simulink model "controller_stateflow"  (R2022b)
settings: Solver=FixedStepAuto  StartTime=0.0  StopTime=inf  FixedStep=0.05  RelTol=1e-3
PreLoadFcn:
  | rosinit();
model workspace (MAT data in the model file):
  SL_ROS_VariableLengthArrays_MaxSizes : object (value not decoded)
  pitch = -10
  restart = 0
undefined symbols (not defined in the file): StartTime
libraries: robotmaniplib x62, robotlib x17, robotcorelib x4, robotgazebolib x1
(part 2 of 4)

== system controller_stateflow/Summit Controller Command ==
  time : Inport
  sum_cntr : Inport  Port=2
  Enable : EnablePort
  Blank Message4 : robotlib/Blank Message  messageClass=Message  entityType=geometry_msgs/Twist  messageType=geometry_msgs/Twist  SampleTime=inf  legacyBusStruct=off
  Publish : robotlib/Publish  topicSource=Select from ROS network  topic=/robotnik_base_control/cmd_vel  messageType=geometry_msgs/Twist  legacyBusStruct=off  messageQueueLength=1
  summit_VelocityController_command : MATLAB Function  TreatAsAtomicUnit=on
  wires:
  Blank Message4/1 -> summit_VelocityController_command/2(msgIn)
  summit_VelocityController_command/1(msgOut) -> Publish/1
  time/1 -> summit_VelocityController_command/1(Time)
  sum_cntr/1 -> summit_VelocityController_command/3(sum_cntr)

== system controller_stateflow/UR10e Controller Command ==
  time : Inport
  TimeFromStart : Inport  Port=2
  Point_array : Inport  Port=3
  Enable : EnablePort
  Blank Message : robotlib/Blank Message  messageClass=Message  entityType=trajectory_msgs/JointTrajectory  messageType=trajectory_msgs/JointTrajectory  SampleTime=inf  legacyBusStruct=off
  Blank Message1 : robotlib/Blank Message  messageClass=Message  entityType=trajectory_msgs/JointTrajectoryPoint  messageType=trajectory_msgs/JointTrajectoryPoint  SampleTime=inf  legacyBusStruct=off
  Publish : robotlib/Publish  topicSource=Select from ROS network  topic=/ur10e_eff_joint_traj_controller/command  messageType=trajectory_msgs/JointTrajectory  legacyBusStruct=off  messageQueueLength=1
  ur10e_TrajectoryController_command : MATLAB Function  TreatAsAtomicUnit=on
  wires:
  Blank Message/1 -> ur10e_TrajectoryController_command/2(msgIn)
  Blank Message1/1 -> ur10e_TrajectoryController_command/3(msgPoint)
  ur10e_TrajectoryController_command/1(msgOut) -> Publish/1
  time/1 -> ur10e_TrajectoryController_command/1(Time)
  TimeFromStart/1 -> ur10e_TrajectoryController_command/4(TimeFromStart)
  Point_array/1 -> ur10e_TrajectoryController_command/5(Point_array)

== matlab function controller_stateflow/General State Flow/get_panda_pose3/MATLAB Function ==
  data: Pose output; boxPos input; boxZYX input; sumPos input; sumZYX input; panda_state input; Weights output; initialGuess output; state input; NWayPoints output; durTime output
function [Pose, Weights, initialGuess, NWayPoints, durTime] = fcn(boxPos,boxZYX,sumPos,sumZYX,panda_state,state)
    
    distance_10 = 0.2;
    distance_10_h = 0.1;

    dimBox   = [0.2;0.2;0.13]; %like a box but we know it's a cilinder
    dimboxUp = [0.23;0.23;0.03]; 
    box_center = [0.115;0.115;0.065]; %to mach the origin of stl with real 3D origin of the cilinder

    toSumChapa = [0;0;0.51];
    toFranka = [0.25;-0.22+0.02;0.15];
    boxPos_offset = [0;0;0];
    
    NWayPoints = 1;
    durTime = 2;
    distance = eye(4,4);
    ZYX_d = [0,0,0];

    Weights = [1,1,1,1,1,1];


    if state == 2
        boxPos_offset = [0;dimBox(2)/2+0.05;+dimBox(3)/2]+box_center;
        ZYX_d = [pi+pi/2,-pi/2,0];
        distance = [[eul2rotm([0,0,0],'ZYX')],[-distance_10,0,0]'; ...
                                0 0 0                       1              ];
        NWayPoints = 1;
        durTime = 2;
    end
    if state == 4
        boxPos_offset = [0;dimBox(2)/2+0.05;+dimBox(3)/2-0.1]+box_center;
        ZYX_d = [pi+pi/2,-pi/2,0];
        distance = [[eul2rotm([0,0,0],'ZYX')],[0,0,0]'; ...
                                0 0 0            1   ];
        NWayPoints = 3;
        durTime = 2;
    end
    if state == 5
        boxPos_offset = [0;dimBox(2)/2;+dimBox(3)/2-0.1]+box_center;
        ZYX_d = [pi+pi/2,-pi/2,0];
        NWayPoints = 5;
        durTime = 2;
    end
    if state == 6
        boxPos_offset = [0;dimBox(2)/2-0.02;+dimBox(3)/2-0.03]+box_center;
        ZYX_d = [pi+pi/2,-pi/2,0];
        NWayPoints = 5;
        durTime = 2;
    end
    if state == 9
        boxPos_offset = [0;dimBox(2)/2;+dimBox(3)/2]+box_center;
        distance = [[eul2rotm([0,0,0],'ZYX')],[-0.15,0,+0.1]'; ...
                        0 0 0            1   ];
        ZYX_d = [pi/2,0,0];
        NWayPoints = 5;
        durTime = 2;
    end
    if state == 11
        boxPos_offset = [0;dimBox(2)/2+0.02;dimBox(3)/2-0.02]+box_center;
        ZYX_d = [pi+pi/2,-pi/16,0];
        boxPos =[1;0;0.65];     %pose in terna summit::base_footprint
        boxZYX =[-pi/2;0;0];
        sumPos = [0;0;0];
        sumZYX = [0;0;0];
        NWayPoints = 5;
        durTime = 5;
    end

    if state == 12
        boxPos_offset = [0;-dimBox(2)/2-0.12;+dimBox(3)/2+0.07]+box_center;
        ZYX_d = [pi/2,-pi/16,0];
        NWayPoints = 5;
        durTime = 5;
    end

    if state == 13
        boxPos_offset = [0;-dimBox(2)/2-0.09;+dimBox(3)/2-0.02]+box_center;
        ZYX_d = [pi/2,-pi/16,0];
        NWayPoints = 5;
        durTime = 5;
    end

    % Trasformazione world -> box::frame
    boxtf_01 = [[eul2rotm(boxZYX', 'ZYX')],boxPos; ...
            0 0 0                               1           ];
    % Trasformazione world -> summit::base_footprint
    sumtf_01 = [[eul2rotm(sumZYX', 'ZYX')],sumPos; ...
                0 0 0                               1           ];
    
    % Trasformazione summit::base_footprint -> panda::base
    sumtopandatf_12 = [[eul2rotm([0,pi/4,0], 'ZYX')],toSumChapa+toFranka; ...
                0 0 0                               1           ];
    
    % Trasformazione world -> panda::base
    toPandatf = sumtf_01*sumtopandatf_12;
    
    % Trasformo la posizione da world frame a panda::base frame per l'IK
    Pose_d0 = boxtf_01*[[eul2rotm(ZYX_d,'ZYX')],[boxPos_offset(1);boxPos_offset(2);boxPos_offset(3)]; ...
                                0 0 0                               1           ];

    Pose = distance*inv(toPandatf)*Pose_d0;

    initialGuess = panda_state;

end

== matlab function controller_stateflow/General State Flow/get_ur_pose_cnvy/MATLAB Function3 ==
  data: u input; y output
function y = fcn(u)

y = u(1:6);

== matlab function controller_stateflow/General State Flow/get_panda_pose3/MATLAB Function4 ==
  data: pose_d input; Pose1 output; T input; Pose2 output; Pose3 output; NWayPoint input; Pose4 output; Pose5 output
function [Pose1,Pose2,Pose3,Pose4,Pose5] = fcn(pose_d,T,NWayPoint)

    coder.extrinsic('slerp');

    if NWayPoint == 1
        Pose1 = pose_d;
        Pose2 = pose_d;
        Pose3 = pose_d;
        Pose4 = pose_d;
        Pose5 = pose_d;
    else

        %semplice interpolazione lineare sulla posizione tra posizione
        %attuale e posizione desiderata
        pos_act   = T(1:3,4);
        pos_d     = pose_d(1:3,4);
        delta_pos = (pos_d-pos_act)/5; 
                  
        q_d = rotm2quat(pose_d(1:3,1:3));
        q_a = rotm2quat(T(1:3,1:3));
        q =   slerp(quaternion(q_a),quaternion(q_d),0:0.2:1);

        Pose1 = [quat2rotm(q(1)),pos_act+delta_pos*1; ...
                 0 0 0                               1           ];
        Pose2 = [quat2rotm(q(2)),pos_act+delta_pos*2; ...
                 0 0 0                               1           ];
        Pose3 = [quat2rotm(q(3)),pos_act+delta_pos*3; ...
                 0 0 0                               1           ];
        Pose4 = [quat2rotm(q(4)),pos_act+delta_pos*4; ...
                 0 0 0                               1           ];

        Pose5 = pose_d;
    end

end

== matlab function controller_stateflow/Wait 0,1 second ==
  data: u input; e output double
function e = wait(u)
% Wait 1e8 nanosecond after start for all Gazebo components starting

    e=0;
    if u.Nsec > 1e8
        e=1;
    end

end

== matlab function controller_stateflow/General State Flow/get_panda_pose3/MATLAB Function6 ==
  data: u input; y output
function y = fcn(u)

y = u(1:7);

== matlab function controller_stateflow/Wait 1 second ==
  data: u input; e output double
function e = wait(u)
% Wait 1 second after start for all Gazebo components starting
    e=0;
    if u.Sec >= 1
        e=1;
    end
end

== matlab function controller_stateflow/Force Generator Function ==
  data: enable output; msgOut output Bus: SL_Bus_controller_stateflow_ApplyBodyWrenchRequest_gxwnto; msgIn input Bus: SL_Bus_controller_stateflow_ApplyBodyWrenchRequest_gxwnto; state input; coll input; T_ur_velvCnt input; pick_type input; state_4_collBox input
function [enable,msgOut]  = force_generator(msgIn,state,coll,T_ur_velvCnt, pick_type, state_4_collBox)

    msgOut = msgIn;
    
    bodyname = 'box_38_18_14::link_0';   % type 1
  
    if pick_type == 1
        bodyname = 'box_38_18_14::link_0';
        else if pick_type == 2
                bodyname = 'box_19_14_29::link_0';
            else if pick_type == 3
                    bodyname = 'cilinder_20_13::link_0';
                else if pick_type == 4 && state_4_collBox == 1
                        bodyname = 'box_38_18_14::link_0';
                    else if pick_type == 4 && state_4_collBox == 2
                        bodyname = 'box_38_18_14_0::link_0';
                    end
                end
            end
        end
    end

    enable = 0;
    
    lenName = uint32(length(bodyname));
    msgOut.BodyName(1:lenName,1) = uint8(convertStringsToChars(bodyname))';
    msgOut.BodyName_SL_Info.CurrentLength = uint32(lenName);
   
    msgOut.ReferenceFrame(1:lenName,1) = uint8(convertStringsToChars(bodyname))';
    msgOut.ReferenceFrame_SL_Info.CurrentLength = uint32(lenName);
    
    msgOut.Wrench.Force.X =  0;
    msgOut.Wrench.Force.Y =  0;
    msgOut.Wrench.Force.Z =  0;
    msgOut.Wrench.Torque.X = 0;
    msgOut.Wrench.Torque.Y = 0;
    msgOut.Wrench.Torque.Z = 0;
        
    F_v = [0;0;0;1];

    if state == 1 && coll == 1
        k=0.75;
%         F_v = [0;0;-80*k;1];
        F_v = [-80*k;0;0;1];

        msgOut.Wrench.Torque.X = 0;
        msgOut.Wrench.Torque.Y = 0;
        msgOut.Wrench.Torque.Z = 0;

        msgOut.ReferencePoint.X = 0;
        msgOut.ReferencePoint.Y = 0;
        msgOut.ReferencePoint.Z = 0;
        
        msgOut.Duration.Sec = 0;
        msgOut.Duration.Nsec = 1e7;

        fprintf("pull \n");

        enable = 1;
    end


    if state == -1
        k=1.0;
%         F_v = [0;0;80*k;1];
        F_v = [80*k;0;0;1];

        msgOut.Wrench.Torque.X = 0;
        msgOut.Wrench.Torque.Y = 0;
        msgOut.Wrench.Torque.Z = 0;
        
        msgOut.ReferencePoint.X = 0;
        msgOut.ReferencePoint.Y = 0;
        msgOut.ReferencePoint.Z = 0;

        msgOut.Duration.Sec = 0;
        msgOut.Duration.Nsec = 1e7;

        fprintf("push \n");

        enable = 1;        
    end
        
    F_w = T_ur_velvCnt*F_v;

    msgOut.Wrench.Force.X = F_w(1);
    msgOut.Wrench.Force.Y = F_w(2);
    msgOut.Wrench.Force.Z = F_w(3);

end

== matlab function controller_stateflow/UR10e Controller Command/ur10e_TrajectoryController_command ==
  data: Time input; msgOut output Bus: SL_Bus_controller_stateflow_trajectory_msgs_JointTrajectory; msgIn input; msgPoint input; TimeFromStart input; Point_array input
function msgOut   = ur10e_TrajectoryController_command(Time, msgIn, msgPoint,TimeFromStart, Point_array)
% In this function we create the TrajecotryJointController message for the
% ROS topic to command movements of manipulator.
    msgOut = msgIn;
    if Time.Sec ~= 0

        jointNames = {'ur10e_shoulder_pan_joint','ur10e_shoulder_lift_joint','ur10e_elbow_joint'...
            'ur10e_wrist_1_joint','ur10e_wrist_2_joint','ur10e_wrist_3_joint'};
        numJoints = uint32(length(jointNames));
        msgOut.JointNames_SL_Info.CurrentLength = numJoints;
        for idx = 1:numJoints
            jName = jointNames{idx};
            lenName = uint32(length(jName));
            msgOut.JointNames(idx).Data(1:lenName) = uint8(jName);
            msgOut.JointNames(idx).Data_SL_Info.CurrentLength = lenName;
        end

        msgOut.Header.Stamp.Sec = Time.Sec;
        msgOut.Header.Stamp.Nsec = Time.Nsec;
        
        msgOut.Header.Seq = uint32(0);
        
        %if the points are all equals, the command is to reach that point
        %in one pooint position command, in TimeFromStart time.
        if isequal(Point_array(:,1),Point_array(:,2))
            msgOut.Points_SL_Info.CurrentLength = uint32(1);
            msgOut.Points(1) = msgPoint;
            msgOut.Points(1).Positions(1:6) = Point_array(1:6,1);
            msgOut.Points(1).Positions_SL_Info.CurrentLength = uint32(6);
            msgOut.Points(1).TimeFromStart.Sec = TimeFromStart;
            msgOut.Points(1).TimeFromStart.Nsec = 0;
        else
            % otherwise the command is a trajectory command and the time is
            % divided for each point.
            msgOut.Points_SL_Info.CurrentLength = uint32(size(Point_array,2));
                
            for i = 1:size(Point_array,2)
                msgOut.Points(i) = msgPoint;
                msgOut.Points(i).Positions(1:6) = Point_array(1:6,i);
                msgOut.Points(i).Positions_SL_Info.CurrentLength = uint32(6);

                msgOut.Points(i).TimeFromStart.Sec = TimeFromStart + 1*i;
                msgOut.Points(i).TimeFromStart.Nsec = 0;

                time = TimeFromStart*1e9;
                time_i_nsec = time/5*i;
                msgOut.Points(i).TimeFromStart.Sec = fix(time_i_nsec/1e9);
                msgOut.Points(i).TimeFromStart.Nsec = time_i_nsec-fix(time_i_nsec/1e9);
            end
        end
        
    end
end

== matlab function controller_stateflow/General State Flow/get_panda_pose_cnvy/MATLAB Function ==
  data: Pose output; boxPos input; boxZYX input; sumPos input; sumZYX input; panda_state input; data input; Weights output; initialGuess output; state input; NWayPoints output; durTime output
function [Pose, Weights, initialGuess, NWayPoints, durTime] = fcn(boxPos,boxZYX,sumPos,sumZYX,panda_state,data, state)
    
    distance_10 = 0.2;
    distance_10_h = 0.1;
    dimBox=[0.38,0.18,0.14];
    toSumChapa = [0;0;0.51];
    toFranka = [0.25;-0.22+0.02;0.15];
    boxPos_offset = [0;0;0];
    
    NWayPoints = 1;
    durTime = 2;
    distance = eye(4,4);
    ZYX_d = [0,0,0];

    Weights = [1,1,1,1,1,1];


%     % Trasformazione world -> box::frame
%     boxtf_01 = [[eul2rotm(boxZYX', 'ZYX')],boxPos; ...
%             0 0 0                               1           ];
%     % Trasformazione world -> summit::base_footprint
%     sumtf_01 = [[eul2rotm(sumZYX', 'ZYX')],sumPos; ...
%                 0 0 0                               1           ];
%     
%     % Trasformazione summit::base_footprint -> panda::base
%     sumtopandatf_12 = [[eul2rotm([0,pi/4,0], 'ZYX')],toSumChapa+toFranka; ...
%                 0 0 0                               1           ];
%     
%     % Trasformazione world -> panda::base
%     toPandatf = sumtf_01*sumtopandatf_12;
%     
%     % Trasformo la posizione da world frame a panda::base frame per l'IK
%     Pose_d0 = boxtf_01*[[eul2rotm(ZYX_d,'ZYX')],[boxPos_offset(1);boxPos_offset(2);boxPos_offset(3)]; ...
%                                 0 0 0                               1           ];
% 
%     Pose = distance*inv(toPandatf)*Pose_d0;

    Pose = data + [0 0 0 0; 0 0 0 0;0 0 0 0.2;0 0 0 0];     

    initialGuess = panda_state;

end

== matlab function controller_stateflow/Collision Check/MATLAB Function4 ==
  data: x output; T input; T_end input; y output; box_pos input; box_ZYX input; box2_pos input; box2_ZYX input; z output; sumPos input; sumZYX input; T_ur_velvCnt output; coll output; boxx output; pick_type input; state_4_collBox input
function [x,y,z,T_ur_velvCnt,coll,boxx] = collision_fnc(T,T_end,box_pos,box_ZYX,box2_pos,box2_ZYX,sumPos,sumZYX,pick_type,state_4_collBox)
    
    dimBox = [0;0;0];
    box = box_pos;
    boxZYX = box_ZYX;

    % Based on the pick_type, choose the right dimensions of the box
    if pick_type == 1 || pick_type == 4
        dimBox = [0.38;0.18;0.14];
        else if pick_type == 2
                dimBox=[0.19,0.14,0.29];
            else if pick_type == 3
                    dimBox = [0.2;0.2;0.13];
                    box_center = [0.115;0.115;0.065]; %to mach the origin of stl with real 3D origin of the cilinder
            end
        end
    end
    
    if pick_type == 4 && state_4_collBox == 1
        box = box_pos;
        boxZYX = box_ZYX;
    end
    if pick_type == 4 && state_4_collBox == 2
        box = box2_pos;
        boxZYX = box2_ZYX;
    end


    toSumChapa = [0;0;0.51];
    toUR10e = [0.35;0.32;0.05];
    
    velvet_length = 0.28+0.04;
    velvet_height = 0.08;
    
    base_ur_offset = [0;0;0.05];
    
    %Compute the transformation matrix from origin world to velvet
    %center
    sumtf_01 = [[eul2rotm(sumZYX', 'ZYX')],sumPos; ...
                0 0 0                               1           ];
    sumtoUR10etf_12 = [[eul2rotm([0,0,0], 'ZYX')],toSumChapa+toUR10e+base_ur_offset; ...
                0 0 0                               1           ];
    
    toUR10etf = sumtf_01*sumtoUR10etf_12;
    
    
    to_velvCnt = [[eul2rotm([0,0,0], 'ZYX')],[velvet_length-dimBox(2)/2;0;velvet_height/2+dimBox(3)/2]; ...
     0 0 0                               1           ];
    
    T_ur_velvCnt = toUR10etf*T*to_velvCnt;
    
    % compute the distance between the box center and the box center
    boxx = inv(T_ur_velvCnt)*[box;1];
    
    x = boxx(1);
    y = boxx(2);
    z = boxx(3);
    
    coll = 0;
    
    goal = [0.165;0;0];
    tol = [0;0.05;0.05];
    
    if boxx(1) <= goal(1) - tol(1) && ...
       boxx(2) <= goal(2) + tol(2) && boxx(2) >= goal(2) - tol(2) && ...
       boxx(3) <= goal(3) + tol(3) && boxx(3) >= goal(3) - tol(3)
            coll = 1;
    end
  
    

    if pick_type == 3
        box_center = [0.115;0.115;0.065]; %to mach the origin of stl with real 3D origin of the cilinder
        boxPos = box_pos;
        boxPos_offset = [0;0;-dimBox(3)/2]+box_center;

        % trasformation matrix world -> box::frame
        boxtf_01 = [[eul2rotm(boxZYX', 'ZYX')],boxPos; ...
                    0 0 0                               1           ];
        Point_d0 = boxtf_01*[[eul2rotm([0,0,0],'ZYX')],[boxPos_offset(1);boxPos_offset(2);boxPos_offset(3)]; ...
                                0 0 0                               1           ];

        toSumChapa = [0;0;0.51];
        toUR10e = [0.35;0.32;0.05];
        
        velvet_length = 0.28+0.04;
        velvet_height = 0.08;

        %Compute the transformation matrix from origin world to velvet end
        base_ur_offset = [0;0;0.05];
        
        sumtf_01 = [[eul2rotm(sumZYX', 'ZYX')],sumPos; ...
                    0 0 0                               1           ];
        sumtoUR10etf_12 = [[eul2rotm([0,0,0], 'ZYX')],toSumChapa+toUR10e+base_ur_offset; ...
                    0 0 0                               1           ];
        
        toUR10etf = sumtf_01*sumtoUR10etf_12;
        
        T_ur_velv_end = toUR10etf*T_end;

        % compute the distance between the box center and the box center
        boxx = inv(T_ur_velv_end)*Point_d0(1:4,4);

        x = boxx(1);
        y = boxx(2);
        z = boxx(3);
        
        coll = 0;
        
        goal = [0.0;0;0];
        tol = [0.01;0.05;0.05];
        
        if boxx(1) <= goal(1) + tol(1) && ...
           boxx(2) <= goal(2) + tol(2) && boxx(2) >= goal(2) - tol(2) && ...
           boxx(3) <= goal(3) + tol(3) && boxx(3) >= goal(3) - tol(3)
                coll = 1;
        end
    end

end

== matlab function controller_stateflow/Collision Check/MATLAB Function6 ==
  data: u input; y output
function y = fcn(u)

y = u(1:6);

== matlab function controller_stateflow/Collision Check/MATLAB Function7 ==
  data: box_ok output; x input; y input; z input; box_off output; pick_type input
function [box_ok,box_off]  = box_on_off(x,y,z,pick_type)

    box_ok = 0;
    box_off = 0;

    if  x <= -0.01
        box_ok=1;
    end

    if  x >= 0.17
        box_off=1;
    end

    if pick_type == 3

        box_ok = 0;
        box_off = 0;
    
        if  x <= -0.10
            box_ok=1;
        end
    
        if  x >= 0.02
            box_off=1;
        end
    end


end

== matlab function controller_stateflow/General State Flow/get_ur_pose/MATLAB Function4 ==
  data: pose_d input; Pose1 output; T input; Pose2 output; Pose3 output; NWayPoint input; Pose4 output; Pose5 output
function [Pose1,Pose2,Pose3,Pose4,Pose5] = fcn(pose_d,T,NWayPoint)

    coder.extrinsic('slerp');

    if NWayPoint == 1
        Pose1 = pose_d;
        Pose2 = pose_d;
        Pose3 = pose_d;
        Pose4 = pose_d;
        Pose5 = pose_d;
    else

        %semplice interpolazione lineare sulla posizione tra posizione
        %attuale e posizione desiderata
        pos_act   = T(1:3,4);
        pos_d     = pose_d(1:3,4);
        delta_pos = (pos_d-pos_act)/5; 
                  
        q_d = rotm2quat(pose_d(1:3,1:3));
        q_a = rotm2quat(T(1:3,1:3));
        q =   slerp(quaternion(q_a),quaternion(q_d),0:0.2:1);

        Pose1 = [quat2rotm(q(1)),pos_act+delta_pos*1; ...
                 0 0 0                               1           ];
        Pose2 = [quat2rotm(q(2)),pos_act+delta_pos*2; ...
                 0 0 0                               1           ];
        Pose3 = [quat2rotm(q(3)),pos_act+delta_pos*3; ...
                 0 0 0                               1           ];
        Pose4 = [quat2rotm(q(4)),pos_act+delta_pos*4; ...
                 0 0 0                               1           ];

        Pose5 = pose_d;
    end

end

== matlab function controller_stateflow/General State Flow/get_ur_pose/MATLAB Function6 ==
  data: u input; y output
function y = fcn(u)

y = u(1:6);

== matlab function controller_stateflow/General State Flow/get_panda_pose_cnvy/MATLAB Function4 ==
  data: pose_d input; Pose1 output; T input; Pose2 output; Pose3 output; NWayPoint input; Pose4 output; Pose5 output
function [Pose1,Pose2,Pose3,Pose4,Pose5] = fcn(pose_d,T,NWayPoint)

    coder.extrinsic('slerp');

    if NWayPoint == 1
        Pose1 = pose_d;
        Pose2 = pose_d;
        Pose3 = pose_d;
        Pose4 = pose_d;
        Pose5 = pose_d;
    else

        %semplice interpolazione lineare sulla posizione tra posizione
        %attuale e posizione desiderata
        pos_act   = T(1:3,4);
        pos_d     = pose_d(1:3,4);
        delta_pos = (pos_d-pos_act)/5; 
                  
        q_d = rotm2quat(pose_d(1:3,1:3));
        q_a = rotm2quat(T(1:3,1:3));
        q =   slerp(quaternion(q_a),quaternion(q_d),0:0.2:1);

        Pose1 = [quat2rotm(q(1)),pos_act+delta_pos*1; ...
                 0 0 0                               1           ];
        Pose2 = [quat2rotm(q(2)),pos_act+delta_pos*2; ...
                 0 0 0                               1           ];
        Pose3 = [quat2rotm(q(3)),pos_act+delta_pos*3; ...
                 0 0 0                               1           ];
        Pose4 = [quat2rotm(q(4)),pos_act+delta_pos*4; ...
                 0 0 0                               1           ];

        Pose5 = pose_d;
    end

end

== matlab function controller_stateflow/General State Flow/get_panda_pose_cnvy/MATLAB Function6 ==
  data: u input; y output
function y = fcn(u)

y = u(1:7);

== matlab function controller_stateflow/General State Flow/get_panda_pose/MATLAB Function4 ==
  data: pose_d input; Pose1 output; T input; Pose2 output; Pose3 output; NWayPoint input; Pose4 output; Pose5 output
function [Pose1,Pose2,Pose3,Pose4,Pose5] = fcn(pose_d,T,NWayPoint)

    coder.extrinsic('slerp');

    if NWayPoint == 1
        Pose1 = pose_d;
        Pose2 = pose_d;
        Pose3 = pose_d;
        Pose4 = pose_d;
        Pose5 = pose_d;
    else

        %semplice interpolazione lineare sulla posizione tra posizione
        %attuale e posizione desiderata
        pos_act   = T(1:3,4);
        pos_d     = pose_d(1:3,4);
        delta_pos = (pos_d-pos_act)/5; 
                  
        q_d = rotm2quat(pose_d(1:3,1:3));
        q_a = rotm2quat(T(1:3,1:3));
        q =   slerp(quaternion(q_a),quaternion(q_d),0:0.2:1);

        Pose1 = [quat2rotm(q(1)),pos_act+delta_pos*1; ...
                 0 0 0                               1           ];
        Pose2 = [quat2rotm(q(2)),pos_act+delta_pos*2; ...
                 0 0 0                               1           ];
        Pose3 = [quat2rotm(q(3)),pos_act+delta_pos*3; ...
                 0 0 0                               1           ];
        Pose4 = [quat2rotm(q(4)),pos_act+delta_pos*4; ...
                 0 0 0                               1           ];

        Pose5 = pose_d;
    end

end

== matlab function controller_stateflow/General State Flow/get_panda_pose/MATLAB Function6 ==
  data: u input; y output
function y = fcn(u)

y = u(1:7);

== matlab function controller_stateflow/General State Flow/get_panda_pose2/MATLAB Function ==
  data: Pose output; boxPos input; boxZYX input; sumPos input; sumZYX input; panda_state input; Weights output; initialGuess output; state input; NWayPoints output; durTime output
function [Pose, Weights, initialGuess, NWayPoints, durTime] = fcn(boxPos,boxZYX,sumPos,sumZYX,panda_state,state)
    
    distance_10 = 0.2;
    distance_10_h = 0.1;

    dimBox=[0.19,0.14,0.29];

    toSumChapa = [0;0;0.51];
    toFranka = [0.25;-0.22+0.02;0.15];
    boxPos_offset = [0;0;0];
    
    NWayPoints = 1;
    durTime = 2;
    distance = eye(4,4);
    ZYX_d = [0,0,0];

    Weights = [1,1,1,1,1,1];

    if state == 2
        boxPos_offset = [0;dimBox(2)/2;+dimBox(3)/2];
        ZYX_d = [pi+pi/2,0,0];
        distance = [[eul2rotm([0,0,0],'ZYX')],[-distance_10-0.1,0,distance_10_h]'; ...
                                0 0 0                       1              ];
        NWayPoints = 1;
        durTime = 2;
    end

    if state == 4
        boxPos_offset = [0;dimBox(2)/2+0.07;dimBox(3)/2-0.02];
        ZYX_d = [pi+pi/2,-pi/8,0];
        NWayPoints = 1;
        durTime = 2;
    end
    if state == 5
        boxPos_offset = [0;dimBox(2)/2;dimBox(3)/2-0.02];
        ZYX_d = [pi+pi/2,-pi/8,0];
        NWayPoints = 1;
        durTime = 2;
    end
    if state == 6
        boxPos_offset = [0;-0.05;dimBox(3)/2];
        ZYX_d = [pi+pi/2,-pi/4,0];
        NWayPoints = 1;
        durTime = 2;
    end
    if state == 7
        boxPos_offset = [0;dimBox(2)/2+0.1;+dimBox(3)/2-0.09];
        ZYX_d = [pi+pi/2,-pi/2-pi/16,0];
        NWayPoints = 1;
        durTime = 2;
    end    
    if state == 8
        boxPos_offset = [0;dimBox(2)/2+0.02;-dimBox(3)/2-0.05];
        ZYX_d = [pi+pi/2,-pi/2-pi/16,0];
        NWayPoints = 1;
        durTime = 2;
    end
    if state == 9
        boxPos_offset = [0;dimBox(2)/2-0.03;-dimBox(3)/2-0.05];
        ZYX_d = [pi+pi/2,-pi/2-pi/16,0];
        NWayPoints = 1;
        durTime = 2;
    end

    if state == 10
        boxPos_offset = [0;dimBox(2)/2-0.05;-dimBox(3)/2+0.05];
        ZYX_d = [pi+pi/2,-pi/2-pi/16,0];
        NWayPoints = 5;
        durTime = 5;
    end
    if state == 11
        boxPos_offset = [0;dimBox(2)/2;-dimBox(3)/2-0.05];
        ZYX_d = [pi+pi/2,-pi/2-pi/8,0];
        NWayPoints = 5;
        durTime = 5;
    end
    
    % Trasformazione world -> box::frame
    boxtf_01 = [[eul2rotm(boxZYX', 'ZYX')],boxPos; ...
            0 0 0                               1           ];
    % Trasformazione world -> summit::base_footprint
    sumtf_01 = [[eul2rotm(sumZYX', 'ZYX')],sumPos; ...
                0 0 0                               1           ];
    
    % Trasformazione summit::base_footprint -> panda::base
    sumtopandatf_12 = [[eul2rotm([0,pi/4,0], 'ZYX')],toSumChapa+toFranka; ...
                0 0 0                               1           ];
    
    % Trasformazione world -> panda::base
    toPandatf = sumtf_01*sumtopandatf_12;
    
    % Trasformo la posizione da world frame a panda::base frame per l'IK
    Pose_d0 = boxtf_01*[[eul2rotm(ZYX_d,'ZYX')],[boxPos_offset(1);boxPos_offset(2);boxPos_offset(3)]; ...
                                0 0 0                               1           ];

    Pose = distance*inv(toPandatf)*Pose_d0;

    initialGuess = panda_state;

end

== matlab function controller_stateflow/General State Flow/get_panda_pose2/MATLAB Function4 ==
  data: pose_d input; Pose1 output; T input; Pose2 output; Pose3 output; NWayPoint input; Pose4 output; Pose5 output
function [Pose1,Pose2,Pose3,Pose4,Pose5] = fcn(pose_d,T,NWayPoint)

    coder.extrinsic('slerp');

    if NWayPoint == 1
        Pose1 = pose_d;
        Pose2 = pose_d;
        Pose3 = pose_d;
        Pose4 = pose_d;
        Pose5 = pose_d;
    else

        %semplice interpolazione lineare sulla posizione tra posizione
        %attuale e posizione desiderata
        pos_act   = T(1:3,4);
        pos_d     = pose_d(1:3,4);
        delta_pos = (pos_d-pos_act)/5; 
                  
        q_d = rotm2quat(pose_d(1:3,1:3));
        q_a = rotm2quat(T(1:3,1:3));
        q =   slerp(quaternion(q_a),quaternion(q_d),0:0.2:1);

        Pose1 = [quat2rotm(q(1)),pos_act+delta_pos*1; ...
                 0 0 0                               1           ];
        Pose2 = [quat2rotm(q(2)),pos_act+delta_pos*2; ...
                 0 0 0                               1           ];
        Pose3 = [quat2rotm(q(3)),pos_act+delta_pos*3; ...
                 0 0 0                               1           ];
        Pose4 = [quat2rotm(q(4)),pos_act+delta_pos*4; ...
                 0 0 0                               1           ];

        Pose5 = pose_d;
    end

end

== matlab function controller_stateflow/General State Flow/get_panda_pose2/MATLAB Function6 ==
  data: u input; y output
function y = fcn(u)

y = u(1:7);

== matlab function controller_stateflow/General State Flow/get_ur_pose2/MATLAB Function ==
  data: Pose output; boxPos input; boxZYX input; sumPos input; sumZYX input; urState input; Weights output; initialGuess output; state input; NWayPoints output; durTime output; T input
function [Pose, Weights, initialGuess, NWayPoints, durTime] = fcn(boxPos,boxZYX,sumPos,sumZYX,urState,state,T)

distance_10 = 0.2;
dimBox=[0.19,0.14,0.29];
toSumChapa = [0;0;0.51];
toUR10e = [0.35;0.32+0.02;0.05];
base_ur_offset = [0;0;0.035];

NWayPoints = 1;
durTime = 2;
distance = eye(4,4);
boxPos_offset = [0;0;0];
ZYX_d = [0,0,0];

% in base allo stato in cui si trovano, definisco punto in cui deve andare
% l'end-effector relativamente alla scatola,l'orientazione dell'ee, la 
% distanza da tale punto, il modo e il tempo
if state == 2
    boxPos_offset = [0;-dimBox(2)/2;-dimBox(3)/2];
    ZYX_d = [pi/2,pi/4,0];
    distance = [[eul2rotm([0,0,0],'ZYX')],[-distance_10,0,0]'; ...
                       0 0 0              1   ];
    NWayPoints = 1;
    durTime = 2;
end

% trasformazione world -> box::frame
boxtf_01 = [[eul2rotm(boxZYX', 'ZYX')],boxPos; ...
            0 0 0                               1           ];

% Trasformazione world -> summit::base_footprint
sumtf_01 = [[eul2rotm(sumZYX', 'ZYX')],sumPos; ...
            0 0 0                               1           ];
% Trasformazione summit::base_footprint -> UR10e::base
sumtoUR10etf_12 = [[eul2rotm([0,0,0], 'ZYX')],toSumChapa+toUR10e+base_ur_offset; ...
            0 0 0                               1           ];
% Trasformazione world -> UR10e::base
toUR10etf = sumtf_01*sumtoUR10etf_12;

% Trasformo la posa da world frame a UR10e::base_frame per l'IK
Point_d0 = boxtf_01*[[eul2rotm(ZYX_d,'ZYX')],[boxPos_offset(1);boxPos_offset(2);boxPos_offset(3)]; ...
                                0 0 0                               1           ];

Pose = distance*inv(toUR10etf)*Point_d0;

if state == 10
    Pose = [  eye(3,3),   [T(1:3,4)]; ...
            0 0 0     1     ];
    NWayPoints = 5;
    durTime = 5;
end

Weights = [1,1,1,1,1,1];
initialGuess = urState(1:6,1);

end

== matlab function controller_stateflow/General State Flow/get_ur_pose2/MATLAB Function4 ==
  data: pose_d input; Pose1 output; T input; Pose2 output; Pose3 output; NWayPoint input; Pose4 output; Pose5 output
function [Pose1,Pose2,Pose3,Pose4,Pose5] = fcn(pose_d,T,NWayPoint)

    coder.extrinsic('slerp');

    if NWayPoint == 1
        Pose1 = pose_d;
        Pose2 = pose_d;
        Pose3 = pose_d;
        Pose4 = pose_d;
        Pose5 = pose_d;
    else

        %semplice interpolazione lineare sulla posizione tra posizione
        %attuale e posizione desiderata
        pos_act   = T(1:3,4);
        pos_d     = pose_d(1:3,4);
        delta_pos = (pos_d-pos_act)/5; 
                  
        q_d = rotm2quat(pose_d(1:3,1:3));
        q_a = rotm2quat(T(1:3,1:3));
        q =   slerp(quaternion(q_a),quaternion(q_d),0:0.2:1);

        Pose1 = [quat2rotm(q(1)),pos_act+delta_pos*1; ...
                 0 0 0                               1           ];
        Pose2 = [quat2rotm(q(2)),pos_act+delta_pos*2; ...
                 0 0 0                               1           ];
        Pose3 = [quat2rotm(q(3)),pos_act+delta_pos*3; ...
                 0 0 0                               1           ];
        Pose4 = [quat2rotm(q(4)),pos_act+delta_pos*4; ...
                 0 0 0                               1           ];

        Pose5 = pose_d;
    end

end

== matlab function controller_stateflow/General State Flow/get_ur_pose2/MATLAB Function6 ==
  data: u input; y output
function y = fcn(u)

y = u(1:6);

== matlab function controller_stateflow/General State Flow/get_ur_pose3/MATLAB Function ==
  data: Pose output; boxPos input; boxZYX input; sumPos input; sumZYX input; urState input; Weights output; initialGuess output; state input; NWayPoints output; durTime output; T input
function [Pose, Weights, initialGuess, NWayPoints, durTime] = fcn(boxPos,boxZYX,sumPos,sumZYX,urState,state,T)

distance_10 = 0.2;
dimBox   = [0.2;0.2;0.13]; %like a box but we know it's a cilinder
dimboxUp = [0.23;0.23;0.03]; 
box_center = [0.115;0.115;0.065]; %to mach the origin of stl with real 3D origin of the cilinder


toSumChapa = [0;0;0.51];
toUR10e = [0.35;0.32+0.04;0.05];
toUR10e = [0.35;0.32;0.05];
base_ur_offset = [0;0;0.035];

NWayPoints = 1;
durTime = 2;
distance = eye(4,4);
boxPos_offset = [0;0;0];
ZYX_d = [0,0,0];

% in base allo stato in cui si trovano, definisco punto in cui deve andare
% l'end-effector relativamente alla scatola,l'orientazione dell'ee, la 
% distanza da tale punto, il modo e il tempo
if state == 2
    boxPos_offset = [0;dimBox(2)/2;-dimBox(3)/2]+box_center;
    ZYX_d = [-pi/2,0,0];
    distance = [[eul2rotm([0,0,0],'ZYX')],[-distance_10-0.05,0,0]'; ...
                       0 0 0              1   ];
    NWayPoints = 1;
    durTime = 2;
end
if state == 4
    boxPos_offset = [0;dimBox(2)/2+0.05;-dimBox(3)/2]+box_center;
    ZYX_d = [-pi/2,0,0];
    distance = [[eul2rotm([0,0,0],'ZYX')],[0,0,0]'; ...
                       0 0 0              1   ];
    NWayPoints = 1;
    durTime = 2;
end

if state == 7
    boxPos_offset = [0;dimBox(2)/2+0.05;-dimBox(3)/2-0.0]+box_center;
    ZYX_d = [-pi/2,0,0];
    NWayPoints = 5;
    durTime = 3;
end

if state == 8
    boxPos_offset = [0;0;-dimBox(3)/2-0.0]+box_center;
    ZYX_d = [-pi/2,0,0];
    NWayPoints = 1;
    durTime = 3;
end

if state == 11
    boxPos_offset = [0;+dimBox(2)/2;-dimBox(3)/2]+box_center;
    ZYX_d = [pi/2,0,0];
    boxPos =[1;0;0.65];     %pose in terna summit::base_footprint
    boxZYX =[-pi/2;0;0];
    sumPos = [0;0;0];
    sumZYX = [0;0;0];
    NWayPoints = 5;
    durTime = 3;
end


% trasformazione world -> box::frame
boxtf_01 = [[eul2rotm(boxZYX', 'ZYX')],boxPos; ...
            0 0 0                               1           ];

% Trasformazione world -> summit::base_footprint
sumtf_01 = [[eul2rotm(sumZYX', 'ZYX')],sumPos; ...
            0 0 0                               1           ];
% Trasformazione summit::base_footprint -> UR10e::base
sumtoUR10etf_12 = [[eul2rotm([0,0,0], 'ZYX')],toSumChapa+toUR10e+base_ur_offset; ...
            0 0 0                               1           ];
% Trasformazione world -> UR10e::base
toUR10etf = sumtf_01*sumtoUR10etf_12;

% Trasformo la posa da world frame a UR10e::base_frame per l'IK
Point_d0 = boxtf_01*[[eul2rotm(ZYX_d,'ZYX')],[boxPos_offset(1);boxPos_offset(2);boxPos_offset(3)]; ...
                                0 0 0                               1           ];

Pose = distance*inv(toUR10etf)*Point_d0;

Weights = [1,1,1,1,1,1];
initialGuess = urState(1:6,1);

end

== matlab function controller_stateflow/General State Flow/get_ur_pose3/MATLAB Function4 ==
  data: pose_d input; Pose1 output; T input; Pose2 output; Pose3 output; NWayPoint input; Pose4 output; Pose5 output
function [Pose1,Pose2,Pose3,Pose4,Pose5] = fcn(pose_d,T,NWayPoint)

    coder.extrinsic('slerp');

    if NWayPoint == 1
        Pose1 = pose_d;
        Pose2 = pose_d;
        Pose3 = pose_d;
        Pose4 = pose_d;
        Pose5 = pose_d;
    else

        %semplice interpolazione lineare sulla posizione tra posizione
        %attuale e posizione desiderata
        pos_act   = T(1:3,4);
        pos_d     = pose_d(1:3,4);
        delta_pos = (pos_d-pos_act)/5; 
                  
        q_d = rotm2quat(pose_d(1:3,1:3));
        q_a = rotm2quat(T(1:3,1:3));
        q =   slerp(quaternion(q_a),quaternion(q_d),0:0.2:1);

        Pose1 = [quat2rotm(q(1)),pos_act+delta_pos*1; ...
                 0 0 0                               1           ];
        Pose2 = [quat2rotm(q(2)),pos_act+delta_pos*2; ...
                 0 0 0                               1           ];
        Pose3 = [quat2rotm(q(3)),pos_act+delta_pos*3; ...
                 0 0 0                               1           ];
        Pose4 = [quat2rotm(q(4)),pos_act+delta_pos*4; ...
                 0 0 0                               1           ];

        Pose5 = pose_d;
    end

end

== matlab function controller_stateflow/General State Flow/get_ur_pose3/MATLAB Function6 ==
  data: u input; y output
function y = fcn(u)

y = u(1:6);

== matlab function controller_stateflow/General State Flow/get_ur_pose4/MATLAB Function ==
  data: Pose output; boxPos input; boxZYX input; boxPos2 input size=[3,1]; boxZYX2 input size=[3,1]; sumPos input; sumZYX input; urState input; Weights output; initialGuess output; state input; NWayPoints output; durTime output
function [Pose, Weights, initialGuess, NWayPoints, durTime] = fcn(boxPos,boxZYX,boxPos2,boxZYX2,sumPos,sumZYX,urState,state)

distance_10 = 0.2;
dimBox=[0.38,0.18,0.14];
toSumChapa = [0;0;0.51];
toUR10e = [0.35;0.32+0.04;0.05];
base_ur_offset = [0;0;0.035];

NWayPoints = 1;
durTime = 2;
distance = eye(4,4);
boxPos_offset = [0;0;0];
ZYX_d = [0,0,0];
box_sel = 1;

% in base allo stato in cui si trovano, definisco punto in cui deve andare
% l'end-effector relativamente alla scatola,l'orientazione dell'ee, la 
% distanza da tale punto, il modo e il tempo
if state == 101
    box_sel = 2;
    boxPos_offset = [-dimBox(1)/2-0.05;dimBox(2)/2;0];
    ZYX_d = [pi/2,0,pi/2];
    distance = [[eul2rotm([0,0,0],'ZYX')],[-distance_10,0,0]'; ...
                       0 0 0              1   ];
    NWayPoints = 1;
    durTime = 2;
end

if state == 111
    box_sel = 2;
    boxPos_offset = [-dimBox(1)/2-0.01;dimBox(2)/2;0];
    ZYX_d = [pi/2,0,pi/2];
    NWayPoints = 1;
    durTime = 2;
end

if state == 131
    box_sel = 2;
    boxPos_offset = [-dimBox(1)/2-0.05;dimBox(2)/2-0.25;0];
    ZYX_d = [pi/2,0,pi/2];
    NWayPoints = 1;
    durTime = 2;
end


if state == 102
    box_sel = 2;
    boxPos_offset = [-dimBox(1)/2-0.05;dimBox(2)/2-0.03;0];
    ZYX_d = [pi/2,0,pi/2];
    distance = [[eul2rotm([0,0,0],'ZYX')],[-distance_10,0,0]'; ...
                       0 0 0              1   ];
    NWayPoints = 1;
    durTime = 2;
end

if state == 112
    box_sel = 2;
    boxPos_offset = [-dimBox(1)/2-0.01;dimBox(2)/2-0.03;0];
    ZYX_d = [pi/2,0,pi/2];
    NWayPoints = 1;
    durTime = 2;
end

if state == 122
    box_sel = 2;
    boxPos_offset = [-dimBox(1)/2-0.01;dimBox(2)/2-0.03;0];
    ZYX_d = [pi/2-pi/8,0,pi/2];
    NWayPoints = 5;
    durTime = 5;
end

if state == 132
    box_sel = 2;
    boxPos_offset = [-dimBox(1)/2-0.1;dimBox(2)/2-0.1;0];
    ZYX_d = [pi/2,0,pi/2];
    NWayPoints = 1;
    durTime = 2;
end


if box_sel == 1
    % trasformazione world -> box1::frame
    boxtf_01 = [[eul2rotm(boxZYX', 'ZYX')],boxPos; ...
                  0 0 0                               1           ];
else % trasformazione world -> box2::frame
    boxtf_01 = [[eul2rotm(boxZYX2', 'ZYX')],boxPos2; ...
                  0 0 0                               1           ];
end

% Trasformazione world -> summit::base_footprint
sumtf_01 = [[eul2rotm(sumZYX', 'ZYX')],sumPos; ...
            0 0 0                               1           ];
% Trasformazione summit::base_footprint -> UR10e::base
sumtoUR10etf_12 = [[eul2rotm([0,0,0], 'ZYX')],toSumChapa+toUR10e+base_ur_offset; ...
            0 0 0                               1           ];
% Trasformazione world -> UR10e::base
toUR10etf = sumtf_01*sumtoUR10etf_12;

% Trasformo la posa da world frame a UR10e::base frame per l'IK
Point_d0 = boxtf_01*[[eul2rotm(ZYX_d,'ZYX')],[boxPos_offset(1);boxPos_offset(2);boxPos_offset(3)]; ...
                                0 0 0                               1           ];


Pose = distance*inv(toUR10etf)*Point_d0;

Weights = [1,1,1,1,1,1];
initialGuess = urState(1:6,1);

end

== matlab function controller_stateflow/General State Flow/get_ur_pose4/MATLAB Function4 ==
  data: pose_d input; Pose1 output; T input; Pose2 output; Pose3 output; NWayPoint input; Pose4 output; Pose5 output
function [Pose1,Pose2,Pose3,Pose4,Pose5] = fcn(pose_d,T,NWayPoint)

    coder.extrinsic('slerp');

    if NWayPoint == 1
        Pose1 = pose_d;
        Pose2 = pose_d;
        Pose3 = pose_d;
        Pose4 = pose_d;
        Pose5 = pose_d;
    else

        %semplice interpolazione lineare sulla posizione tra posizione
        %attuale e posizione desiderata
        pos_act   = T(1:3,4);
        pos_d     = pose_d(1:3,4);
        delta_pos = (pos_d-pos_act)/5; 
                  
        q_d = rotm2quat(pose_d(1:3,1:3));
        q_a = rotm2quat(T(1:3,1:3));
        q =   slerp(quaternion(q_a),quaternion(q_d),0:0.2:1);

        Pose1 = [quat2rotm(q(1)),pos_act+delta_pos*1; ...
                 0 0 0                               1           ];
        Pose2 = [quat2rotm(q(2)),pos_act+delta_pos*2; ...
                 0 0 0                               1           ];
        Pose3 = [quat2rotm(q(3)),pos_act+delta_pos*3; ...
                 0 0 0                               1           ];
        Pose4 = [quat2rotm(q(4)),pos_act+delta_pos*4; ...
                 0 0 0                               1           ];

        Pose5 = pose_d;
    end

end

== matlab function controller_stateflow/General State Flow/get_ur_pose4/MATLAB Function6 ==
  data: u input; y output
function y = fcn(u)

y = u(1:6);

== matlab function controller_stateflow/General State Flow/get_panda_pose4/MATLAB Function ==
  data: Pose output; boxPos input; boxZYX input; boxPos2 input; boxZYX2 input; sumPos input; sumZYX input; panda_state input; Weights output; initialGuess output; state input; NWayPoints output; durTime output
function [Pose, Weights, initialGuess, NWayPoints, durTime] = fcn(boxPos,boxZYX,boxPos2,boxZYX2,sumPos,sumZYX,panda_state,state)
    
    distance_10 = 0.2;
    distance_10_h = 0.1;
    dimBox=[0.38,0.18,0.14];
    toSumChapa = [0;0;0.51];
    toFranka = [0.25;-0.22+0.02;0.15];
    boxPos_offset = [0;0;0];
    
    NWayPoints = 1;
    durTime = 2;
    distance = eye(4,4);
    ZYX_d = [0,0,0];

    Weights = [1,1,1,1,1,1];
    box_sel = 1;

    if state == 101
        boxPos_offset = [dimBox(1)/2+0.05;dimBox(2)/2-0.2;0];
        ZYX_d = [pi+pi/2,0,-pi/2];
        %distance = [[eul2rotm([0,0,0],'ZYX')],[-distance_10,0,0]'; ...
         %                       0 0 0                       1              ];
        NWayPoints = 1;
        durTime = 2;
    end
    if state == 111
        boxPos_offset = [dimBox(1)/2-0.05;dimBox(2)/2;0];
        ZYX_d = [pi+pi/2,0,-pi/2];
        NWayPoints = 5;
        durTime = 2;
    end

    if state == 121
        boxPos_offset = [dimBox(1)/2-0.04;dimBox(2)/2-0.12;0];
        ZYX_d = [pi+pi/2,0,-pi/2];
        NWayPoints = 5;
        durTime = 2;
    end
    if state == 131
        boxPos_offset = [dimBox(1)/2+0.05;dimBox(2)/2;0.3];
        ZYX_d = [pi+pi/2,0,-pi/2];
        NWayPoints = 5;
        durTime = 2;
    end

    if state == 102
        box_sel = 2;
        boxPos_offset = [dimBox(1)/2+0.05;dimBox(2)/2-0.2;0];
        ZYX_d = [pi+pi/2,0,-pi/2];
        %distance = [[eul2rotm([0,0,0],'ZYX')],[-distance_10,0,0]'; ...
         %                       0 0 0                       1              ];
        NWayPoints = 1;
        durTime = 2;
    end
    if state == 112
        box_sel = 2;
        boxPos_offset = [dimBox(1)/2-0.05;dimBox(2)/2;0];
        ZYX_d = [pi+pi/2,0,-pi/2];
        NWayPoints = 1;
        durTime = 2;
    end
    if state == 122
        box_sel = 2;
        boxPos_offset = [dimBox(1)/2-0.03;dimBox(2)/2-0.13;0];
        ZYX_d = [pi+pi/2-pi/8,0,-pi/2];
        NWayPoints = 5;
        durTime = 5;
    end
    if state == 132
        box_sel = 2;
        boxPos_offset = [dimBox(1)/2+0.05;dimBox(2)/2;0.3];
        ZYX_d = [pi+pi/2,0,-pi/2];
        NWayPoints = 1;
        durTime = 2;
    end
    
    if box_sel == 1
        % trasformazione world -> box1::frame
        boxtf_01 = [[eul2rotm(boxZYX', 'ZYX')],boxPos; ...
                      0 0 0                               1           ];
    else % trasformazione world -> box2::frame
        boxtf_01 = [[eul2rotm(boxZYX2', 'ZYX')],boxPos2; ...
                      0 0 0                               1           ];
    end

    % Trasformazione world -> summit::base_footprint
    sumtf_01 = [[eul2rotm(sumZYX', 'ZYX')],sumPos; ...
                0 0 0                               1           ];
    
    % Trasformazione summit::base_footprint -> panda::base
    sumtopandatf_12 = [[eul2rotm([0,pi/4,0], 'ZYX')],toSumChapa+toFranka; ...
                0 0 0                               1           ];
    
    % Trasformazione world -> panda::base
    toPandatf = sumtf_01*sumtopandatf_12;
    
    % Trasformo la posizione da world frame a panda::base frame per l'IK
    Pose_d0 = boxtf_01*[[eul2rotm(ZYX_d,'ZYX')],[boxPos_offset(1);boxPos_offset(2);boxPos_offset(3)]; ...
                                0 0 0                               1           ];

    Pose = inv(toPandatf)*distance*Pose_d0;

    initialGuess = panda_state;

end

== matlab function controller_stateflow/General State Flow/get_panda_pose4/MATLAB Function4 ==
  data: pose_d input; Pose1 output; T input; Pose2 output; Pose3 output; NWayPoint input; Pose4 output; Pose5 output
function [Pose1,Pose2,Pose3,Pose4,Pose5] = fcn(pose_d,T,NWayPoint)

    coder.extrinsic('slerp');

    if NWayPoint == 1
        Pose1 = pose_d;
        Pose2 = pose_d;
        Pose3 = pose_d;
        Pose4 = pose_d;
        Pose5 = pose_d;
    else

        %semplice interpolazione lineare sulla posizione tra posizione
        %attuale e posizione desiderata
        pos_act   = T(1:3,4);
        pos_d     = pose_d(1:3,4);
        delta_pos = (pos_d-pos_act)/5; 
                  
        q_d = rotm2quat(pose_d(1:3,1:3));
        q_a = rotm2quat(T(1:3,1:3));
        q =   slerp(quaternion(q_a),quaternion(q_d),0:0.2:1);

        Pose1 = [quat2rotm(q(1)),pos_act+delta_pos*1; ...
                 0 0 0                               1           ];
        Pose2 = [quat2rotm(q(2)),pos_act+delta_pos*2; ...
                 0 0 0                               1           ];
        Pose3 = [quat2rotm(q(3)),pos_act+delta_pos*3; ...
                 0 0 0                               1           ];
        Pose4 = [quat2rotm(q(4)),pos_act+delta_pos*4; ...
                 0 0 0                               1           ];

        Pose5 = pose_d;
    end

end

== matlab function controller_stateflow/General State Flow/get_panda_pose4/MATLAB Function6 ==
  data: u input; y output
function y = fcn(u)

y = u(1:7);
